simulink model "multi_module_phase_shift_generator_built_in_pwm"  (R2025b)
settings: Solver=VariableStepAuto  StartTime=0.0  StopTime=10.0  RelTol=1e-3
libraries: simulink x3
settings Model: Creator=KoayXianCong  LastModifiedBy=KoayXianCong

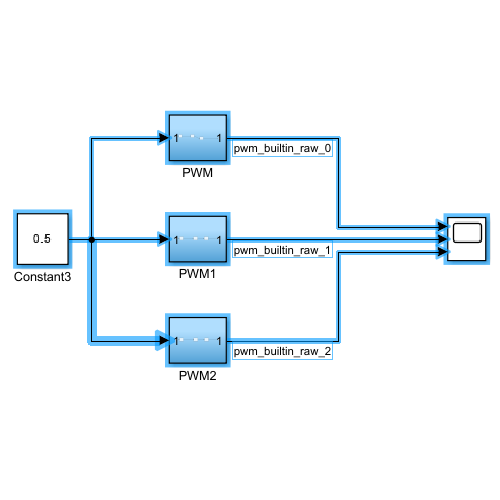
[thumbnail: Simulink's stored preview of the top-level diagram]
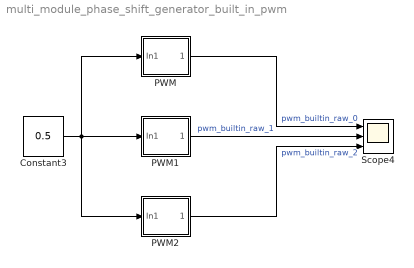
== system multi_module_phase_shift_generator_built_in_pwm ==
  Constant3 : Constant  Value=0.5  VectorParams1D=off  OutDataTypeStr=fixdt(0,16,16)  SampleTime=1
  PWM : Subsystem  Tag=DecoupledSystem
  PWM1 : Subsystem  Tag=DecoupledSystem
  PWM2 : Subsystem  Tag=DecoupledSystem
  Scope4 : Scope  NumInputPorts=3
      settings: ActiveDisplayYMinimum=-0.15719261881639313  ActiveDisplayYMaximum=1.3621901936836069  DataLoggingVariableName=ScopeData4  DataLoggingSaveFormat=Array
  wires:
  PWM/1(Out1) -> Scope4/1  "pwm_builtin_raw_0"
  PWM1/1(Out1) -> Scope4/2  "pwm_builtin_raw_1"
  PWM2/1(Out1) -> Scope4/3  "pwm_builtin_raw_2"
  Constant3/1 -> PWM2/1(In1), PWM/1(In1), PWM1/1(In1)

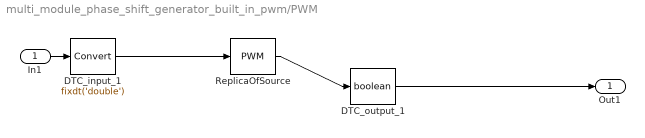
== system multi_module_phase_shift_generator_built_in_pwm/PWM ==
  In1 : Inport  LockScale=on
  DTC_input_1 : DataTypeConversion  OutDataTypeStr=fixdt('double')  RndMeth=Nearest  SaturateOnIntegerOverflow=off  LockScale=on
  DTC_output_1 : DataTypeConversion  OutDataTypeStr=boolean  SaturateOnIntegerOverflow=off  RndMeth=Floor
  ReplicaOfSource : simulink/Discontinuities/PWM  DisableCoverage=on  Period=1024  InitialDelay=0  DisallowZeroDutyCycle=on  RunAtFixedTimeIntervals=on  SampleTime=1
      settings: LibrarySourceBlock=hdlsllib/RCP and HIL/PWM
  Out1 : Outport  LockScale=on
  wires:
  In1/1 -> DTC_input_1/1
  DTC_output_1/1 -> Out1/1
  DTC_input_1/1 -> ReplicaOfSource/1
  ReplicaOfSource/1 -> DTC_output_1/1

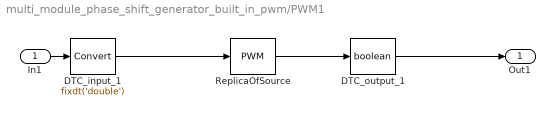
== system multi_module_phase_shift_generator_built_in_pwm/PWM1 ==
  In1 : Inport  LockScale=on
  DTC_input_1 : DataTypeConversion  OutDataTypeStr=fixdt('double')  RndMeth=Nearest  SaturateOnIntegerOverflow=off  LockScale=on
  DTC_output_1 : DataTypeConversion  OutDataTypeStr=boolean  SaturateOnIntegerOverflow=off  RndMeth=Floor
  ReplicaOfSource : simulink/Discontinuities/PWM  DisableCoverage=on  Period=1024  InitialDelay=1024/3  DisallowZeroDutyCycle=on  RunAtFixedTimeIntervals=on  SampleTime=1
      settings: LibrarySourceBlock=hdlsllib/RCP and HIL/PWM
  Out1 : Outport  LockScale=on
  wires:
  ReplicaOfSource/1 -> DTC_output_1/1
  In1/1 -> DTC_input_1/1
  DTC_input_1/1 -> ReplicaOfSource/1
  DTC_output_1/1 -> Out1/1

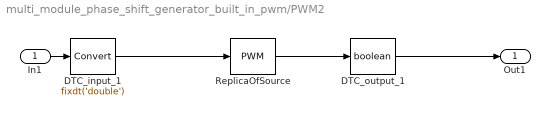
== system multi_module_phase_shift_generator_built_in_pwm/PWM2 ==
  In1 : Inport  LockScale=on
  DTC_input_1 : DataTypeConversion  OutDataTypeStr=fixdt('double')  RndMeth=Nearest  SaturateOnIntegerOverflow=off  LockScale=on
  DTC_output_1 : DataTypeConversion  OutDataTypeStr=boolean  SaturateOnIntegerOverflow=off  RndMeth=Floor
  ReplicaOfSource : simulink/Discontinuities/PWM  DisableCoverage=on  Period=1024  InitialDelay=(2*1024)/3  DisallowZeroDutyCycle=off  RunAtFixedTimeIntervals=on  SampleTime=1
      settings: LibrarySourceBlock=hdlsllib/RCP and HIL/PWM
  Out1 : Outport  LockScale=on
  wires:
  In1/1 -> DTC_input_1/1
  DTC_input_1/1 -> ReplicaOfSource/1
  ReplicaOfSource/1 -> DTC_output_1/1
  DTC_output_1/1 -> Out1/1
